simulink model "task3"  (R2024a)
settings: Solver=VariableStepAuto  StartTime=0.0  StopTime=100  RelTol=1e-3
undefined symbols (not defined in the file): A_m, discr_sys_1, discr_sys_2, init_1, init_2, omega, T_1, T_2
settings Model: Creator=vladislav  LastModifiedBy=vladislav

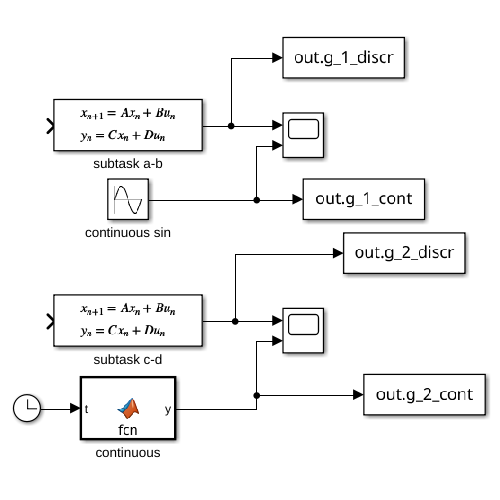
[thumbnail: Simulink's stored preview of the top-level diagram]
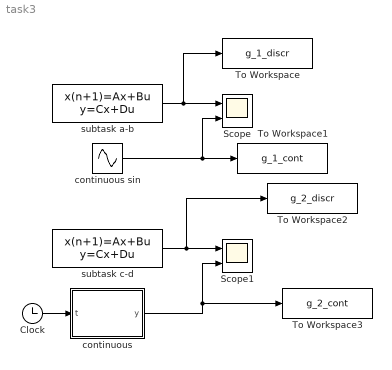
== system task3 ==
  Clock : Clock
  Scope : Scope  NumInputPorts=2
  Scope1 : Scope  NumInputPorts=2
  To Workspace : ToWorkspace  VariableName=g_1_discr  SaveFormat=Timeseries  SampleTime=-1
  To Workspace1 : ToWorkspace  VariableName=g_1_cont  SaveFormat=Timeseries  SampleTime=-1
  To Workspace2 : ToWorkspace  VariableName=g_2_discr  SaveFormat=Timeseries  SampleTime=-1
  To Workspace3 : ToWorkspace  VariableName=g_2_cont  SaveFormat=Timeseries  SampleTime=-1
  continuous : MATLAB Function  TreatAsAtomicUnit=on
  continuous sin : Sin  Amplitude=A_m  Frequency=omega  SampleTime=0
  subtask a-b : DiscreteStateSpace  A=discr_sys_1.A  B=discr_sys_1.B  C=discr_sys_1.C  D=discr_sys_1.D  InitialCondition=init_1  SampleTime=T_1
  subtask c-d : DiscreteStateSpace  A=discr_sys_2.A  B=discr_sys_2.B  C=discr_sys_2.C  D=discr_sys_2.D  InitialCondition=init_2  SampleTime=T_2
  wires:
  subtask a-b/1 -> To Workspace/1, Scope/1
  continuous sin/1 -> To Workspace1/1, Scope/2
  continuous/1(y) -> To Workspace3/1, Scope1/2
  Clock/1 -> continuous/1(t)
  subtask c-d/1 -> To Workspace2/1, Scope1/1

== matlab function task3/continuous ==
  data: t input; y output
function y = fcn(t)

y = exp(-5*t) * sin(6*t + 2.5) + 0.03*t;
